simulink model "Hand"  (R2023b)
settings: Solver=ode45  StartTime=0.0  StopTime=100  RelTol=1e-3  EnableMultiTasking=on
model workspace (MAT data in the model file):
  InitialAngle = 0
libraries: simulink x22, vrlib x16, sharedtransform x15
(part 1 of 2)
Description:
  | Simulink(R) 3D Animation(TM) - Tutorial #3
  | 
  | Tutorial model to be used for 3D World Editor authoring example in the documentation.
  | After creating the virtual world according to the instructions in the documentation, include the VR block
  | in the model and connect B1, B2 coordinates and S scaling to corresponding nodes in
  | the virtual world.
settings Model: Creator=The MathWorks, Inc.  LastModifiedBy=25168
settings SolverCC: AlgebraicLoopSolver=TrustRegion
settings DataIOCC: LimitDataPoints=on  SaveFormat=Array  SaveOutput=off  SaveTime=off  ReturnWorkspaceOutputs=off  SignalLoggingName=logsOut
settings OptimizationCC: BooleanDataType=off  ExpressionDepthLimit=2147483647  InitFltsAndDblsToZero=on  LifeSpan=inf
settings DebuggingCC: UnderspecifiedInitializationDetection=Classic  MergeDetectMultiDrivingBlocksExec=none  CheckExecutionContextPreStartOutputMsg=on  SignalResolutionControl=TryResolveAllWithWarning  MultiTaskDSMMsg=warning  MultiTaskCondExecSysMsg=none  FcnCallInpInsideContextMsg=warning  UnconnectedInputMsg=warning  UnconnectedOutputMsg=warning  UnconnectedLineMsg=warning  StateNameClashWarn=warning  SymbolicDimsDataTypeCodeGenerationDiagnostic=none  SFUnexpectedBacktrackingDiag=warning  SFNoUnconditionalDefaultTransitionDiag=warning  SFExecutionAtInitializationDiag=none  ArithmeticOperatorsInVariantConditions=warning
settings HardwareCC: ProdBitPerPointer=32  ProdBitPerSizeT=32  ProdBitPerPtrDiffT=32  ProdLargestAtomicFloat=None  ProdIntDivRoundTo=Undefined  ProdEndianess=Unspecified  ProdWordSize=32  ProdHWDeviceType=32-bit Generic  TargetUnknown=on
settings ModelReferenceCC: UpdateModelReferenceTargets=IfOutOfDate  EnableRefExpFcnMdlSchedulingChecks=on  PropagateSignalLabelsOutOfModel=off
settings SFSimCC: SimUseLocalCustomCode=off  CustomCodeUndefinedFunction=UseInterfaceOnly
settings RTWCC: RTWUseLocalCustomCode=off
settings CodeAppCC: StateflowObjectComments=on
settings GRTTargetCC: TargetFcnLib=ansi_tfl_tmw.mat  TargetLangStandard=C89/C90 (ANSI)  CombineOutputUpdateFcns=off  GRTInterface=on
settings ConfigComp: CovMetricSettings=d  CovSaveCumulativeToWorkspaceVar=on  CovSaveSingleToWorkspaceVar=on  CovExternalEMLEnable=off  CovSFcnEnable=off

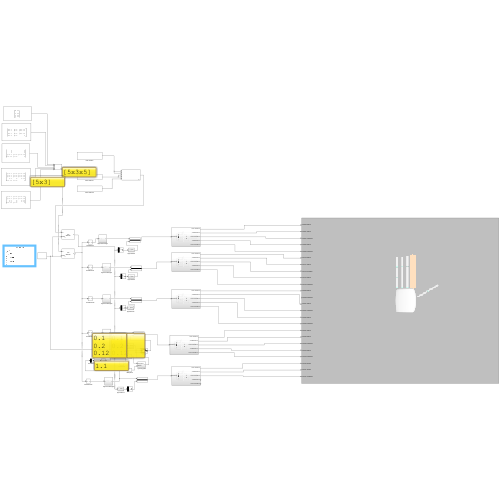
[thumbnail: Simulink's stored preview of the top-level diagram]
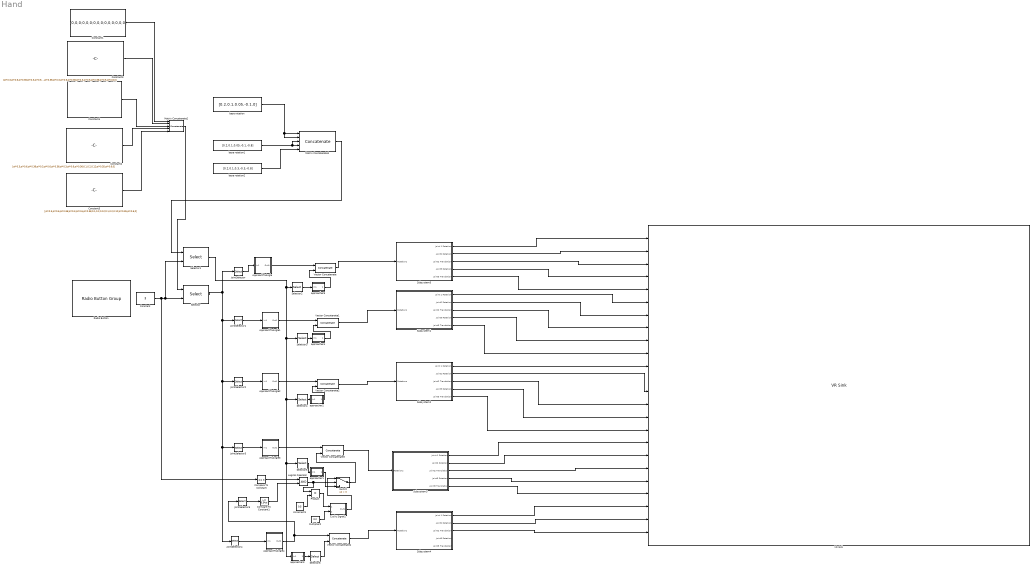
== system Hand ==
  ApproachToAngle : Subsystem
  ApproachToAngle1 : Subsystem
  ApproachToAngle2 : Subsystem
  ApproachToAngle3 : Subsystem
  ApproachToAngle4 : Subsystem
  Compare To Constant : simulink/Logic and Bit Operations/Compare To Constant  relop===  const=3  OutDataTypeStr=boolean
  Compare To Constant1 : simulink/Logic and Bit Operations/Compare To Constant  relop=>=  const=0.3*pi  OutDataTypeStr=boolean
  Constant : Constant  Value=3  VectorParams1D=off
  Constant1 : Constant  Value=[0,0,0;0,0,0;0,0,0;0,0,0;0,0,0]  VectorParams1D=off
  Constant2 : Constant  Value=[pi*0.3,pi*0.6,pi*0.36;pi*0.3,pi*0.6,pi*0.36;pi*0.3,pi*0.6,pi*0.36;0.1,0.2,0.12;pi*0.35,pi*0.6,0]  VectorParams1D=off
  Constant3 : Constant  Value=[pi*0.3,pi*0.6,pi*0.36;pi*0.3,pi*0.6,pi*0.36;pi*0.3,pi*0.6,pi*0.36;pi*0.3,pi*0.6,pi*0.36;pi*0.5,pi*0.8,0]  VectorParams1D=off
  Constant4 : Constant  Value=[0,0,0,;0,0,0;0,0,0;pi*0.1,pi*0.6,pi*0.36;pi*0.35,pi*0.6,0]  VectorParams1D=off
  Constant5 : Constant  Value=[pi*0.3,pi*0.6,pi*0.36;pi*0.3,pi*0.6,pi*0.36;0.1,0.2,0.12;0.1,0.2,0.12;pi*0.35,pi*0.6,0]  VectorParams1D=off
  Cyclic Signal2 : Subsystem
  JointSelector : Selector  NumberOfDimensions=2  IndexMode=Zero-based  InputPortWidth=3  IndexOptions=Index vector (dialog),Select all  Indices=0,0  OutputSizes=1,1
  JointSelector1 : Selector  NumberOfDimensions=2  IndexMode=Zero-based  InputPortWidth=3  IndexOptions=Index vector (dialog),Select all  Indices=1,1  OutputSizes=1,1
  JointSelector2 : Selector  NumberOfDimensions=2  IndexMode=Zero-based  InputPortWidth=3  IndexOptions=Index vector (dialog),Select all  Indices=2,2  OutputSizes=1,1
  JointSelector3 : Selector  NumberOfDimensions=2  IndexMode=Zero-based  InputPortWidth=3  IndexOptions=Index vector (dialog),Select all  Indices=3,2  OutputSizes=1,1
  JointSelector4 : Selector  NumberOfDimensions=2  IndexMode=Zero-based  InputPortWidth=3  IndexOptions=Index vector (dialog),Select all  Indices=4,2  OutputSizes=1,1
  JointSelector5 : Selector  IndexMode=Zero-based  InputPortWidth=3  IndexOptions=Index vector (dialog)  Indices=0  OutputSizes=1
  Logical Operator : Logic  AllPortsSameDT=off  OutDataTypeStr=boolean
  Matrix Concatenate1 : Concatenate  NumInputs=5  Mode=Multidimensional array  ConcatenateDimension=2
  Matrix Concatenate2 : Concatenate  NumInputs=5  Mode=Multidimensional array  ConcatenateDimension=3
  Multiplier2 : Constant  Value=0.2
  Product : Product
  Radio Button : RadioButtonGroup  SelectedLabel=No  ButtonGroupName=Group
      settings: Values={{'Open', 'Close', 'Pinch', 'No', 'V'}, [0 1 2 3 4]}
  Selector : Selector  NumberOfDimensions=3  IndexMode=Zero-based  InputPortWidth=3  IndexOptions=Select all,Select all,Starting index (port)  Indices=[1 3],1,1  OutputSizes=1,1,1
  Selector1 : Selector  NumberOfDimensions=2  IndexMode=Zero-based  InputPortWidth=3  IndexOptions=Select all,Index vector (port)  Indices=[1 3],1  OutputSizes=1,1
  Selector2 : Selector  IndexMode=Zero-based  InputPortWidth=5  IndexOptions=Index vector (dialog)  Indices=0  OutputSizes=1
  Selector3 : Selector  IndexMode=Zero-based  InputPortWidth=5  IndexOptions=Index vector (dialog)  Indices=1  OutputSizes=1
  Selector4 : Selector  IndexMode=Zero-based  InputPortWidth=5  IndexOptions=Index vector (dialog)  Indices=2  OutputSizes=1
  Selector5 : Selector  IndexMode=Zero-based  InputPortWidth=5  IndexOptions=Index vector (dialog)  Indices=3  OutputSizes=1
  Selector6 : Selector  IndexMode=Zero-based  InputPortWidth=5  IndexOptions=Index vector (dialog)  Indices=4  OutputSizes=1
  Subsystem1 : Subsystem
  Subsystem2 : Subsystem
  Subsystem3 : Subsystem
  Subsystem4 : Subsystem
  Subsystem5 : Subsystem
  Switch : Switch  Criteria=u2 > Threshold  ZeroCross=off  SaturateOnIntegerOverflow=off  InputSameDT=off
  VR Sink : vrlib/VR Sink  InstantiateOnLoad=on  SampleTime=0.1  ViewEnable=on  RemoteChange=off  RemoteView=off  FieldsWritten=Joint00.rotation.4.1.1.double#Joint01.rotation.4.1.1.double#Joint01.translation.3.1.1.double#Joint02.rotation.4.1.1.double#Joint02.translation.3.1.1.double#Joint10.rotation.4.1.1.double#Joint11.rotation.4.1.1.double#Joint11.translation.3.1.1.double#Joint12.rotation.4.1.1.double#Joint12.translation.3.1.1.double#Joint20.rotation.4.1.1.double#Joint20.translation.3.1.1.double#Joint21.rotation.4.1.1.double#Joint21.translation.3.1.1.double#Joint22.rotation.4.1.1.double#Joint22.translation.3.1.1.double#Joint31.rotation.4.1.1.double#Joint32.rotation.4.1.1.double#Joint32.translation.3.1.1.double#Joint33.rotation.4.1.1.double#Joint33.translation.3.1.1.double#JointT0.rotation.4.1.1.double#JointT1.rotation.4.1.1.double#JointT1.translation.3.1.1.double  WorldFileName=HW.x3d  AutoView=off  VideoDimensions=[]  AllowVariableSize=off  FigureProperties="{'Position', 'Name', 'Viewpoint', 'CameraBound', 'CameraDirection', 'CameraPosition', 'CameraUpVector', 'ZoomFactor', 'Antialiasing', 'Headlight', 'Lighting', 'NavPanel', 'Sound', 'StatusBar', 'Stereo3D', 'Stereo3DCameraOffset', 'Stereo3DHIT', 'ToolBar', 'Textures', 'Transparency', 'Triad', 'Wireframe', 'NavZones', 'NavMode', 'NavSpeed', 'CaptureFileFormat', 'CaptureFileName', 'Record2DCompressMethod', 'Record2DCompressQuality', 'Record2D', 'Record2DFileName', 'Record2DFPS'; [6.5500000000000000e+02   3.1433333333333337e+02   5.0933333333333326e+02   3.5000000000000000e+02], '', '', 'on', [-4.8608255793823621e-02  -6.0845975116805943e-02  -9.9696289037315999e-01], [9.6584636817473193e+00  -6.5460684286128101e-01   1.1919806951157568e+02], [4.8294533019942611e-02   9.9683214525226260e-01  -6.3192659956020442e-02], [1.0000000000000000e+00], 'on', 'on', 'on', 'halfbar', 'on', 'on', 'off', [1.0000000149011612e-01], [0.0000000000000000e+00], 'on', 'on', 'on', 'none', 'off', 'off', 'examine', 'normal', 'tif', '%f_anim_%n.tif', 'auto', [7.5000000000000000e+01], 'off', '%f_anim_%n.avi', 'auto'}"
  Vector Concatenate{,1..4} (5 alike) : Concatenate
  approacher1 : Subsystem
  approacher2 : Subsystem
  approacher3 : Subsystem
  approacher4 : Subsystem
  approacher5 : Subsystem
  base rotation : Constant  Value=[0.2,0.1,0.05,-0.1,0]
  base rotation1 : Constant  Value=[0.2,0.1,0.05,-0.1,-0.8]
  base rotation2 : Constant  Value=[0.2,0.1,0.3,-0.3,-0.8]
  increment1 : Constant  Value=0.5
  wires:
  Subsystem5/3(Joint2 Translation) -> VR Sink/3
  Subsystem5/4(Joint3 Rotation) -> VR Sink/4
  Subsystem5/1(Joint 1 Rotation) -> VR Sink/1
  Subsystem5/2(Joint2 Rotation) -> VR Sink/2
  Subsystem5/5(Joint3 Translation) -> VR Sink/5
  Subsystem1/1(Joint 1 Rotation) -> VR Sink/6
  Subsystem1/2(Joint2 Rotation) -> VR Sink/7
  Subsystem1/3(Joint2 Translation) -> VR Sink/8
  Subsystem1/4(Joint3 Rotation) -> VR Sink/9
  Subsystem1/5(Joint3 Translation) -> VR Sink/10
  Subsystem4/1(Joint 1 Rotation) -> VR Sink/22
  Subsystem4/2(Joint2 Rotation) -> VR Sink/23
  Subsystem4/3(Joint2 Translation) -> VR Sink/24
  Subsystem2/1(Joint 1 Rotation) -> VR Sink/11
  Subsystem2/2(Joint2 Rotation) -> VR Sink/13
  Subsystem2/3(Joint2 Translation) -> VR Sink/14
  Subsystem2/4(Joint3 Rotation) -> VR Sink/15
  Subsystem2/5(Joint3 Translation) -> VR Sink/16
  Subsystem3/1(Joint 1 Rotation) -> VR Sink/17
  Subsystem3/2(Joint2 Rotation) -> VR Sink/18
  Subsystem3/3(Joint2 Translation) -> VR Sink/19
  Subsystem3/4(Joint3 Rotation) -> VR Sink/20
  Subsystem3/5(Joint3 Translation) -> VR Sink/21
  Constant/1 -> Compare To Constant/1, Selector1/2, Selector/2
  Constant1/1 -> Matrix Concatenate2/1
  Constant2/1 -> Matrix Concatenate2/4
  Constant3/1 -> Matrix Concatenate2/2
  Matrix Concatenate2/1 -> Selector/1
  ApproachToAngle/1(Out1) -> Vector Concatenate/1
  JointSelector/1 -> ApproachToAngle/1(In1)
  JointSelector2/1 -> ApproachToAngle2/1(In1)
  Selector/1 -> JointSelector1/1, JointSelector4/1, JointSelector3/1, JointSelector2/1, JointSelector/1
  Vector Concatenate/1 -> Subsystem5/1(Rotations)
  ApproachToAngle1/1(Out1) -> Vector Concatenate1/1
  JointSelector1/1 -> ApproachToAngle1/1(In1)
  Vector Concatenate1/1 -> Subsystem1/1(Rotations)
  ApproachToAngle2/1(Out1) -> Vector Concatenate2/1
  Selector4/1 -> approacher2/1(In1)
  Vector Concatenate2/1 -> Subsystem2/1(Rotations)
  ApproachToAngle3/1(Out1) -> Vector Concatenate3/1
  JointSelector3/1 -> ApproachToAngle3/1(In1)
  ApproachToAngle4/1(Out1) -> JointSelector5/1, Vector Concatenate4/1
  Selector6/1 -> Vector Concatenate4/2
  JointSelector4/1 -> ApproachToAngle4/1(In1)
  Vector Concatenate4/1 -> Subsystem4/1(Rotations)
  Selector1/1 -> approacher3/1(In1), Selector5/1, Selector4/1, Selector3/1, Selector2/1
  base rotation/1 -> Matrix Concatenate1/2, Matrix Concatenate1/1
  base rotation1/1 -> Matrix Concatenate1/3, Matrix Concatenate1/4
  Constant4/1 -> Matrix Concatenate2/3
  Matrix Concatenate1/1 -> Selector1/1
  Compare To Constant/1 -> Logical Operator/1
  Multiplier2/1 -> Cyclic Signal2/2(Scaler)
  increment1/1 -> Product/2
  Logical Operator/1 -> Product/1, Switch/2
  JointSelector5/1 -> Compare To Constant1/1
  Constant5/1 -> Matrix Concatenate2/5
  Vector Concatenate3/1 -> Subsystem3/1(Rotations)
  Switch/1 -> Vector Concatenate3/2
  Cyclic Signal2/1(Out1) -> Switch/1
  Compare To Constant1/1 -> Logical Operator/2
  Product/1 -> Cyclic Signal2/1(Frequency)
  base rotation2/1 -> Matrix Concatenate1/5
  approacher3/1(Joint 1) -> Selector6/1
  Selector5/1 -> approacher1/1(In1)
  approacher1/1(Joint 1) -> Switch/3
  approacher2/1(Joint 1) -> Vector Concatenate2/2
  Selector3/1 -> approacher4/1(In1)
  approacher4/1(Joint 1) -> Vector Concatenate1/2
  Selector2/1 -> approacher5/1(In1)
  approacher5/1(Joint 1) -> Vector Concatenate/2

== system Hand/ApproachToAngle ==
  In1 : Inport
  Matrix Concatenate1 : Concatenate  NumInputs=3  ConcatenateDimension=2
  Selector1 : Selector  IndexMode=Zero-based  InputPortWidth=3  IndexOptions=Index vector (dialog)  Indices=1  OutputSizes=1
  Selector2 : Selector  IndexMode=Zero-based  InputPortWidth=3  IndexOptions=Index vector (dialog)  Indices=0  OutputSizes=1  RuntimeRangeChecks=on
  Selector3 : Selector  IndexMode=Zero-based  InputPortWidth=3  IndexOptions=Index vector (dialog)  Indices=2  OutputSizes=1
  approacher1 : Subsystem
  approacher2 : Subsystem
  approacher3 : Subsystem
  Out1 : Outport
  wires:
  Selector3/1 -> approacher3/1(In1)
  Selector2/1 -> approacher2/1(In1)
  approacher3/1(Joint 1) -> Matrix Concatenate1/3
  approacher1/1(Joint 1) -> Matrix Concatenate1/2
  approacher2/1(Joint 1) -> Matrix Concatenate1/1
  Selector1/1 -> approacher1/1(In1)
  In1/1 -> Selector3/1, Selector2/1, Selector1/1
  Matrix Concatenate1/1 -> Out1/1

== system Hand/ApproachToAngle1 ==
  In1 : Inport
  Matrix Concatenate1 : Concatenate  NumInputs=3  ConcatenateDimension=2
  Selector1 : Selector  IndexMode=Zero-based  InputPortWidth=3  IndexOptions=Index vector (dialog)  Indices=1  OutputSizes=1
  Selector2 : Selector  IndexMode=Zero-based  InputPortWidth=3  IndexOptions=Index vector (dialog)  Indices=0  OutputSizes=1  RuntimeRangeChecks=on
  Selector3 : Selector  IndexMode=Zero-based  InputPortWidth=3  IndexOptions=Index vector (dialog)  Indices=2  OutputSizes=1
  approacher1 : Subsystem
  approacher2 : Subsystem
  approacher3 : Subsystem
  Out1 : Outport
  wires:
  Selector3/1 -> approacher3/1(In1)
  Selector2/1 -> approacher2/1(In1)
  approacher3/1(Joint 1) -> Matrix Concatenate1/3
  approacher1/1(Joint 1) -> Matrix Concatenate1/2
  approacher2/1(Joint 1) -> Matrix Concatenate1/1
  Selector1/1 -> approacher1/1(In1)
  In1/1 -> Selector3/1, Selector2/1, Selector1/1
  Matrix Concatenate1/1 -> Out1/1

== system Hand/ApproachToAngle2 ==
  In1 : Inport
  Matrix Concatenate1 : Concatenate  NumInputs=3  ConcatenateDimension=2
  Selector1 : Selector  IndexMode=Zero-based  InputPortWidth=3  IndexOptions=Index vector (dialog)  Indices=1  OutputSizes=1
  Selector2 : Selector  IndexMode=Zero-based  InputPortWidth=3  IndexOptions=Index vector (dialog)  Indices=0  OutputSizes=1  RuntimeRangeChecks=on
  Selector3 : Selector  IndexMode=Zero-based  InputPortWidth=3  IndexOptions=Index vector (dialog)  Indices=2  OutputSizes=1
  approacher1 : Subsystem
  approacher2 : Subsystem
  approacher3 : Subsystem
  Out1 : Outport
  wires:
  Selector3/1 -> approacher3/1(In1)
  Selector2/1 -> approacher2/1(In1)
  approacher3/1(Joint 1) -> Matrix Concatenate1/3
  approacher1/1(Joint 1) -> Matrix Concatenate1/2
  approacher2/1(Joint 1) -> Matrix Concatenate1/1
  Selector1/1 -> approacher1/1(In1)
  In1/1 -> Selector3/1, Selector2/1, Selector1/1
  Matrix Concatenate1/1 -> Out1/1

== system Hand/ApproachToAngle3 ==
  In1 : Inport
  Matrix Concatenate1 : Concatenate  NumInputs=3  ConcatenateDimension=2
  Selector1 : Selector  IndexMode=Zero-based  InputPortWidth=3  IndexOptions=Index vector (dialog)  Indices=1  OutputSizes=1
  Selector2 : Selector  IndexMode=Zero-based  InputPortWidth=3  IndexOptions=Index vector (dialog)  Indices=0  OutputSizes=1  RuntimeRangeChecks=on
  Selector3 : Selector  IndexMode=Zero-based  InputPortWidth=3  IndexOptions=Index vector (dialog)  Indices=2  OutputSizes=1
  approacher1 : Subsystem
  approacher2 : Subsystem
  approacher3 : Subsystem
  Out1 : Outport
  wires:
  Selector3/1 -> approacher3/1(In1)
  Selector2/1 -> approacher2/1(In1)
  approacher3/1(Joint 1) -> Matrix Concatenate1/3
  approacher1/1(Joint 1) -> Matrix Concatenate1/2
  approacher2/1(Joint 1) -> Matrix Concatenate1/1
  Selector1/1 -> approacher1/1(In1)
  In1/1 -> Selector3/1, Selector2/1, Selector1/1
  Matrix Concatenate1/1 -> Out1/1

== system Hand/ApproachToAngle4 ==
  In1 : Inport
  Matrix Concatenate1 : Concatenate  NumInputs=3  ConcatenateDimension=2
  Selector1 : Selector  IndexMode=Zero-based  InputPortWidth=3  IndexOptions=Index vector (dialog)  Indices=1  OutputSizes=1
  Selector2 : Selector  IndexMode=Zero-based  InputPortWidth=3  IndexOptions=Index vector (dialog)  Indices=0  OutputSizes=1  RuntimeRangeChecks=on
  Selector3 : Selector  IndexMode=Zero-based  InputPortWidth=3  IndexOptions=Index vector (dialog)  Indices=2  OutputSizes=1
  approacher1 : Subsystem
  approacher2 : Subsystem
  approacher3 : Subsystem
  Out1 : Outport
  wires:
  Selector3/1 -> approacher3/1(In1)
  Selector2/1 -> approacher2/1(In1)
  approacher3/1(Joint 1) -> Matrix Concatenate1/3
  approacher1/1(Joint 1) -> Matrix Concatenate1/2
  approacher2/1(Joint 1) -> Matrix Concatenate1/1
  Selector1/1 -> approacher1/1(In1)
  In1/1 -> Selector3/1, Selector2/1, Selector1/1
  Matrix Concatenate1/1 -> Out1/1

== system Hand/Cyclic Signal2 ==
  Frequency : Inport
  Scaler : Inport  Port=2
  Constant : Constant  Value=pi
  Integrator : Integrator  UpperSaturationLimit=Inf  LowerSaturationLimit=-Inf
  Product : Product
  Product1 : Product
  Trigonometric Function5 : Trigonometry
  Out1 : Outport
  wires:
  Integrator/1 -> Trigonometric Function5/1
  Trigonometric Function5/1 -> Product1/1
  Product1/1 -> Out1/1
  Scaler/1 -> Product1/2
  Frequency/1 -> Product/1
  Constant/1 -> Product/2
  Product/1 -> Integrator/1

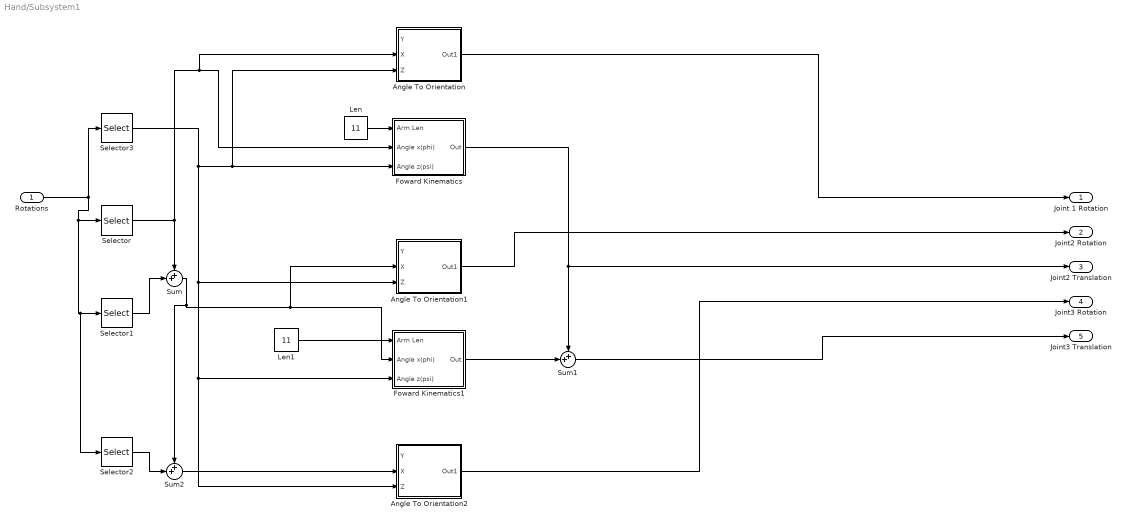
== system Hand/Subsystem1 ==
  Rotations : Inport
  Angle To Orientation : Subsystem
  Angle To Orientation1 : Subsystem
  Angle To Orientation2 : Subsystem
  Foward Kinematics : Subsystem
  Foward Kinematics1 : Subsystem
  Len : Constant  Value=11
  Len1 : Constant  Value=11
  Selector : Selector  InputPortWidth=4  IndexOptions=Index vector (dialog)  Indices=1  OutputSizes=1
  Selector1 : Selector  InputPortWidth=4  IndexOptions=Index vector (dialog)  Indices=2  OutputSizes=1
  Selector2 : Selector  InputPortWidth=4  IndexOptions=Index vector (dialog)  Indices=3  OutputSizes=1
  Selector3 : Selector  InputPortWidth=4  IndexOptions=Index vector (dialog)  Indices=4  OutputSizes=1
  Sum : Sum  Inputs=++|
  Sum1 : Sum  Inputs=++|
  Sum2 : Sum  Inputs=++|
  Joint 1 Rotation : Outport
  Joint2 Rotation : Outport  Port=2
  Joint2 Translation : Outport  Port=3
  Joint3 Rotation : Outport  Port=4
  Joint3 Translation : Outport  Port=5
  wires:
  Foward Kinematics/1(Out) -> Joint2 Translation/1, Sum1/1
  Selector3/1 -> Foward Kinematics1/3(Angle z(psi)), Angle To Orientation2/3(Z), Angle To Orientation1/3(Z), Angle To Orientation/3(Z), Foward Kinematics/3(Angle z(psi))
  Sum2/1 -> Angle To Orientation2/2(X)
  Selector/1 -> Angle To Orientation/2(X), Foward Kinematics/2(Angle x(phi)), Sum/1
  Sum1/1 -> Joint3 Translation/1
  Sum/1 -> Sum2/1, Angle To Orientation1/2(X), Foward Kinematics1/2(Angle x(phi))
  Len/1 -> Foward Kinematics/1(Arm Len)
  Foward Kinematics1/1(Out) -> Sum1/2
  Len1/1 -> Foward Kinematics1/1(Arm Len)
  Angle To Orientation1/1(Out1) -> Joint2 Rotation/1
  Angle To Orientation2/1(Out1) -> Joint3 Rotation/1
  Angle To Orientation/1(Out1) -> Joint 1 Rotation/1
  Selector2/1 -> Sum2/2
  Selector1/1 -> Sum/2
  Rotations/1 -> Selector2/1, Selector1/1, Selector/1, Selector3/1

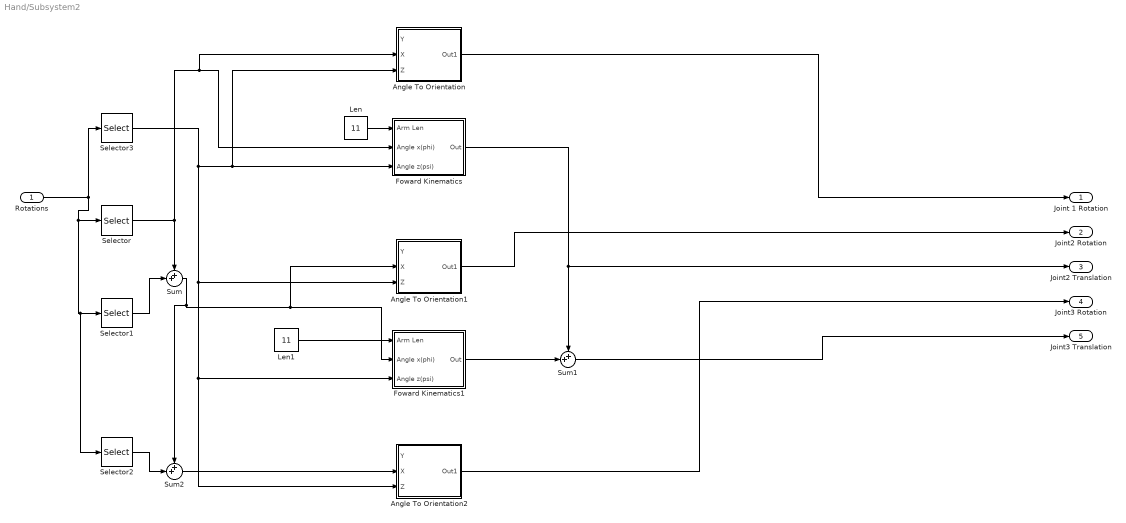
== system Hand/Subsystem2 ==
  Rotations : Inport
  Angle To Orientation : Subsystem
  Angle To Orientation1 : Subsystem
  Angle To Orientation2 : Subsystem
  Foward Kinematics : Subsystem
  Foward Kinematics1 : Subsystem
  Len : Constant  Value=11
  Len1 : Constant  Value=11
  Selector : Selector  InputPortWidth=4  IndexOptions=Index vector (dialog)  Indices=1  OutputSizes=1
  Selector1 : Selector  InputPortWidth=4  IndexOptions=Index vector (dialog)  Indices=2  OutputSizes=1
  Selector2 : Selector  InputPortWidth=4  IndexOptions=Index vector (dialog)  Indices=3  OutputSizes=1
  Selector3 : Selector  InputPortWidth=4  IndexOptions=Index vector (dialog)  Indices=4  OutputSizes=1
  Sum : Sum  Inputs=++|
  Sum1 : Sum  Inputs=++|
  Sum2 : Sum  Inputs=++|
  Joint 1 Rotation : Outport
  Joint2 Rotation : Outport  Port=2
  Joint2 Translation : Outport  Port=3
  Joint3 Rotation : Outport  Port=4
  Joint3 Translation : Outport  Port=5
  wires:
  Foward Kinematics/1(Out) -> Joint2 Translation/1, Sum1/1
  Selector3/1 -> Foward Kinematics1/3(Angle z(psi)), Angle To Orientation2/3(Z), Angle To Orientation1/3(Z), Angle To Orientation/3(Z), Foward Kinematics/3(Angle z(psi))
  Sum2/1 -> Angle To Orientation2/2(X)
  Selector/1 -> Angle To Orientation/2(X), Foward Kinematics/2(Angle x(phi)), Sum/1
  Sum1/1 -> Joint3 Translation/1
  Sum/1 -> Sum2/1, Angle To Orientation1/2(X), Foward Kinematics1/2(Angle x(phi))
  Len/1 -> Foward Kinematics/1(Arm Len)
  Foward Kinematics1/1(Out) -> Sum1/2
  Len1/1 -> Foward Kinematics1/1(Arm Len)
  Angle To Orientation1/1(Out1) -> Joint2 Rotation/1
  Angle To Orientation2/1(Out1) -> Joint3 Rotation/1
  Angle To Orientation/1(Out1) -> Joint 1 Rotation/1
  Selector2/1 -> Sum2/2
  Selector1/1 -> Sum/2
  Rotations/1 -> Selector2/1, Selector1/1, Selector/1, Selector3/1

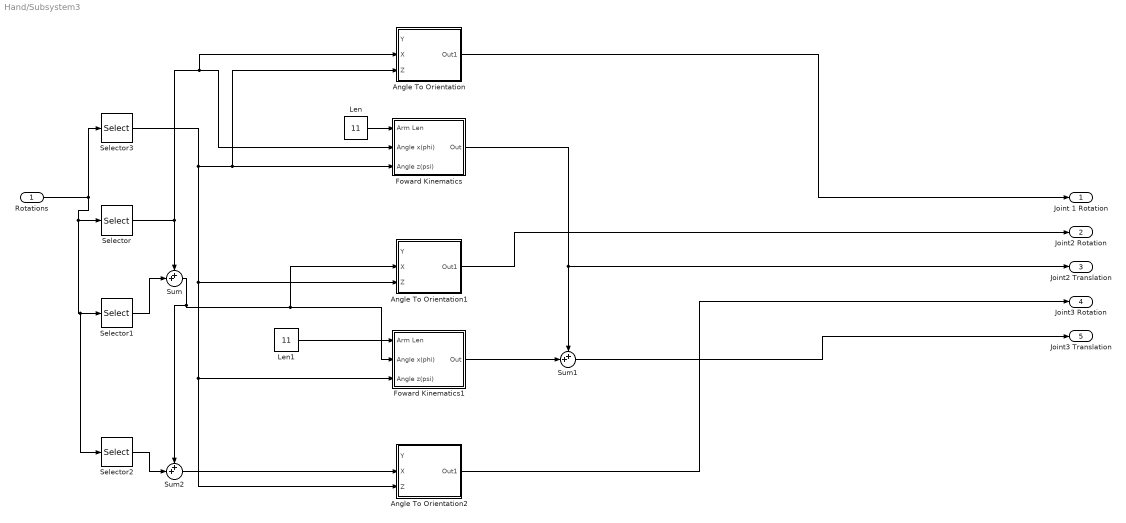
== system Hand/Subsystem3 ==
  Rotations : Inport
  Angle To Orientation : Subsystem
  Angle To Orientation1 : Subsystem
  Angle To Orientation2 : Subsystem
  Foward Kinematics : Subsystem
  Foward Kinematics1 : Subsystem
  Len : Constant  Value=11
  Len1 : Constant  Value=11
  Selector : Selector  InputPortWidth=4  IndexOptions=Index vector (dialog)  Indices=1  OutputSizes=1
  Selector1 : Selector  InputPortWidth=4  IndexOptions=Index vector (dialog)  Indices=2  OutputSizes=1
  Selector2 : Selector  InputPortWidth=4  IndexOptions=Index vector (dialog)  Indices=3  OutputSizes=1
  Selector3 : Selector  InputPortWidth=4  IndexOptions=Index vector (dialog)  Indices=4  OutputSizes=1
  Sum : Sum  Inputs=++|
  Sum1 : Sum  Inputs=++|
  Sum2 : Sum  Inputs=++|
  Joint 1 Rotation : Outport
  Joint2 Rotation : Outport  Port=2
  Joint2 Translation : Outport  Port=3
  Joint3 Rotation : Outport  Port=4
  Joint3 Translation : Outport  Port=5
  wires:
  Foward Kinematics/1(Out) -> Joint2 Translation/1, Sum1/1
  Selector3/1 -> Foward Kinematics1/3(Angle z(psi)), Angle To Orientation2/3(Z), Angle To Orientation1/3(Z), Angle To Orientation/3(Z), Foward Kinematics/3(Angle z(psi))
  Sum2/1 -> Angle To Orientation2/2(X)
  Selector/1 -> Angle To Orientation/2(X), Foward Kinematics/2(Angle x(phi)), Sum/1
  Sum1/1 -> Joint3 Translation/1
  Sum/1 -> Sum2/1, Angle To Orientation1/2(X), Foward Kinematics1/2(Angle x(phi))
  Len/1 -> Foward Kinematics/1(Arm Len)
  Foward Kinematics1/1(Out) -> Sum1/2
  Len1/1 -> Foward Kinematics1/1(Arm Len)
  Angle To Orientation1/1(Out1) -> Joint2 Rotation/1
  Angle To Orientation2/1(Out1) -> Joint3 Rotation/1
  Angle To Orientation/1(Out1) -> Joint 1 Rotation/1
  Selector2/1 -> Sum2/2
  Selector1/1 -> Sum/2
  Rotations/1 -> Selector2/1, Selector1/1, Selector/1, Selector3/1

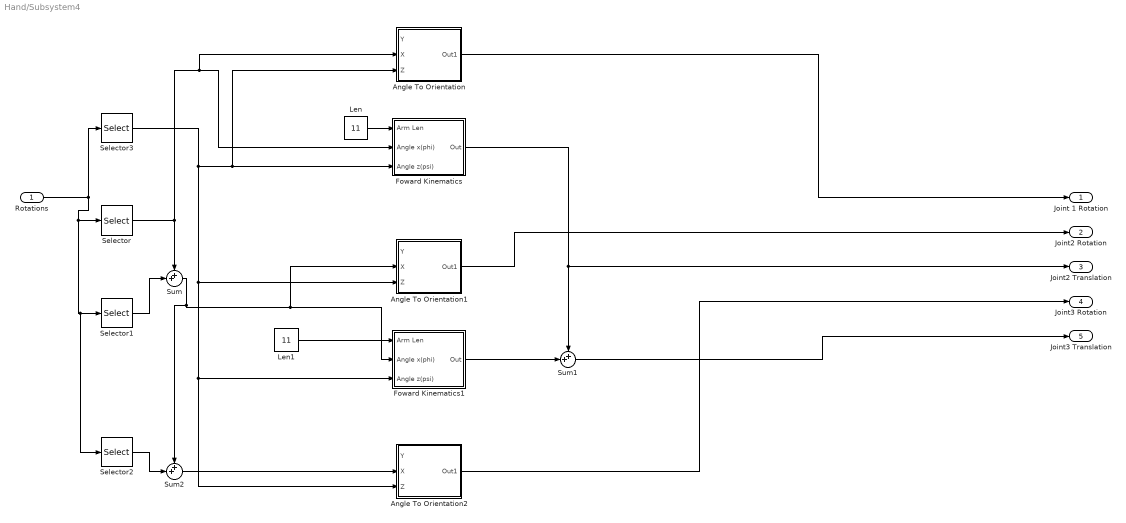
== system Hand/Subsystem4 ==
  Rotations : Inport
  Angle To Orientation : Subsystem
  Angle To Orientation1 : Subsystem
  Angle To Orientation2 : Subsystem
  Foward Kinematics : Subsystem
  Foward Kinematics1 : Subsystem
  Len : Constant  Value=11
  Len1 : Constant  Value=11
  Selector : Selector  InputPortWidth=4  IndexOptions=Index vector (dialog)  Indices=1  OutputSizes=1
  Selector1 : Selector  InputPortWidth=4  IndexOptions=Index vector (dialog)  Indices=2  OutputSizes=1
  Selector2 : Selector  InputPortWidth=4  IndexOptions=Index vector (dialog)  Indices=3  OutputSizes=1
  Selector3 : Selector  InputPortWidth=4  IndexOptions=Index vector (dialog)  Indices=4  OutputSizes=1
  Sum : Sum  Inputs=++|
  Sum1 : Sum  Inputs=++|
  Sum2 : Sum  Inputs=++|
  Joint 1 Rotation : Outport
  Joint2 Rotation : Outport  Port=2
  Joint2 Translation : Outport  Port=3
  Joint3 Rotation : Outport  Port=4
  Joint3 Translation : Outport  Port=5
  wires:
  Foward Kinematics/1(Out) -> Joint2 Translation/1, Sum1/1
  Selector3/1 -> Foward Kinematics1/3(Angle z(psi)), Angle To Orientation2/3(Z), Angle To Orientation1/3(Z), Angle To Orientation/3(Z), Foward Kinematics/3(Angle z(psi))
  Sum2/1 -> Angle To Orientation2/2(X)
  Selector/1 -> Angle To Orientation/2(X), Foward Kinematics/2(Angle x(phi)), Sum/1
  Sum1/1 -> Joint3 Translation/1
  Sum/1 -> Sum2/1, Angle To Orientation1/2(X), Foward Kinematics1/2(Angle x(phi))
  Len/1 -> Foward Kinematics/1(Arm Len)
  Foward Kinematics1/1(Out) -> Sum1/2
  Len1/1 -> Foward Kinematics1/1(Arm Len)
  Angle To Orientation1/1(Out1) -> Joint2 Rotation/1
  Angle To Orientation2/1(Out1) -> Joint3 Rotation/1
  Angle To Orientation/1(Out1) -> Joint 1 Rotation/1
  Selector2/1 -> Sum2/2
  Selector1/1 -> Sum/2
  Rotations/1 -> Selector2/1, Selector1/1, Selector/1, Selector3/1

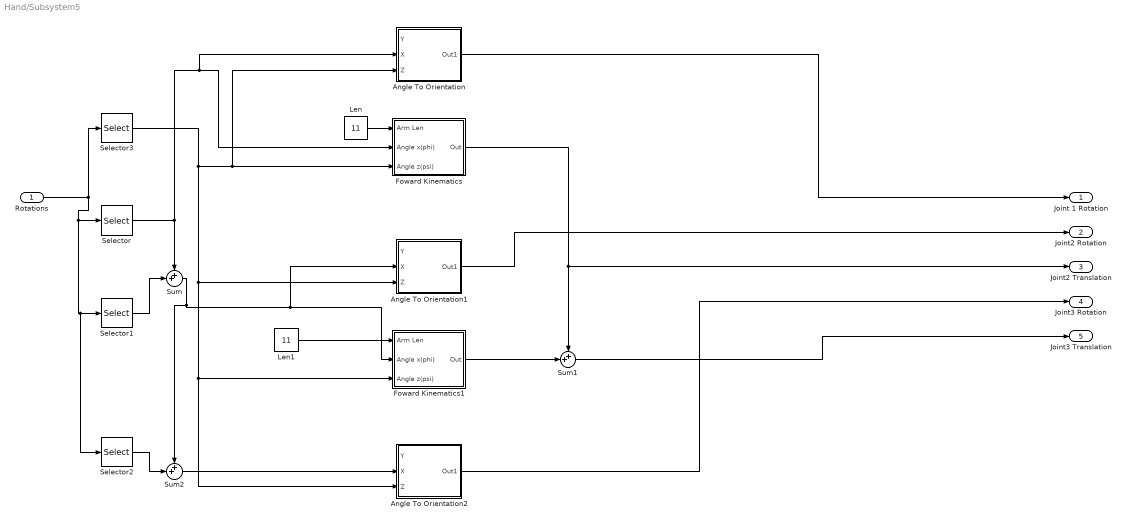
== system Hand/Subsystem5 ==
  Rotations : Inport
  Angle To Orientation : Subsystem
  Angle To Orientation1 : Subsystem
  Angle To Orientation2 : Subsystem
  Foward Kinematics : Subsystem
  Foward Kinematics1 : Subsystem
  Len : Constant  Value=11
  Len1 : Constant  Value=11
  Selector : Selector  InputPortWidth=4  IndexOptions=Index vector (dialog)  Indices=1  OutputSizes=1
  Selector1 : Selector  InputPortWidth=4  IndexOptions=Index vector (dialog)  Indices=2  OutputSizes=1
  Selector2 : Selector  InputPortWidth=4  IndexOptions=Index vector (dialog)  Indices=3  OutputSizes=1
  Selector3 : Selector  InputPortWidth=4  IndexOptions=Index vector (dialog)  Indices=4  OutputSizes=1
  Sum : Sum  Inputs=++|
  Sum1 : Sum  Inputs=++|
  Sum2 : Sum  Inputs=++|
  Joint 1 Rotation : Outport
  Joint2 Rotation : Outport  Port=2
  Joint2 Translation : Outport  Port=3
  Joint3 Rotation : Outport  Port=4
  Joint3 Translation : Outport  Port=5
  wires:
  Foward Kinematics/1(Out) -> Joint2 Translation/1, Sum1/1
  Selector3/1 -> Foward Kinematics1/3(Angle z(psi)), Angle To Orientation2/3(Z), Angle To Orientation1/3(Z), Angle To Orientation/3(Z), Foward Kinematics/3(Angle z(psi))
  Sum2/1 -> Angle To Orientation2/2(X)
  Selector/1 -> Angle To Orientation/2(X), Foward Kinematics/2(Angle x(phi)), Sum/1
  Sum1/1 -> Joint3 Translation/1
  Sum/1 -> Sum2/1, Angle To Orientation1/2(X), Foward Kinematics1/2(Angle x(phi))
  Len/1 -> Foward Kinematics/1(Arm Len)
  Foward Kinematics1/1(Out) -> Sum1/2
  Len1/1 -> Foward Kinematics1/1(Arm Len)
  Angle To Orientation1/1(Out1) -> Joint2 Rotation/1
  Angle To Orientation2/1(Out1) -> Joint3 Rotation/1
  Angle To Orientation/1(Out1) -> Joint 1 Rotation/1
  Selector2/1 -> Sum2/2
  Selector1/1 -> Sum/2
  Rotations/1 -> Selector2/1, Selector1/1, Selector/1, Selector3/1

== system Hand/approacher1 ==
  In1 : Inport
  Compare To Zero : simulink/Logic and Bit Operations/Compare To Zero  relop=<=  OutDataTypeStr=boolean  ZeroCross=off
  Gain : Gain  Gain=-1
  Integrator : Integrator  ZeroCross=off
  Subtract : Sum  Inputs=+-
  Switch : Switch  Criteria=u2 > Threshold  ZeroCross=off  SaturateOnIntegerOverflow=off  InputSameDT=off
  increment : Constant  Value=0.2
  Joint 1 : Outport
  wires:
  Gain/1 -> Switch/3
  Subtract/1 -> Compare To Zero/1
  Compare To Zero/1 -> Switch/2
  Integrator/1 -> Joint 1/1, Subtract/1
  Switch/1 -> Integrator/1
  increment/1 -> Switch/1, Gain/1
  In1/1 -> Subtract/2

== system Hand/approacher2 ==
  In1 : Inport
  Compare To Zero : simulink/Logic and Bit Operations/Compare To Zero  relop=<=  OutDataTypeStr=boolean  ZeroCross=off
  Gain : Gain  Gain=-1
  Integrator : Integrator  ZeroCross=off
  Subtract : Sum  Inputs=+-
  Switch : Switch  Criteria=u2 > Threshold  ZeroCross=off  SaturateOnIntegerOverflow=off  InputSameDT=off
  increment : Constant  Value=0.2
  Joint 1 : Outport
  wires:
  Gain/1 -> Switch/3
  Subtract/1 -> Compare To Zero/1
  Compare To Zero/1 -> Switch/2
  Integrator/1 -> Joint 1/1, Subtract/1
  Switch/1 -> Integrator/1
  increment/1 -> Switch/1, Gain/1
  In1/1 -> Subtract/2

== system Hand/approacher3 ==
  In1 : Inport
  Compare To Zero : simulink/Logic and Bit Operations/Compare To Zero  relop=<=  OutDataTypeStr=boolean  ZeroCross=off
  Gain : Gain  Gain=-1
  Integrator : Integrator  ZeroCross=off
  Subtract : Sum  Inputs=+-
  Switch : Switch  Criteria=u2 > Threshold  ZeroCross=off  SaturateOnIntegerOverflow=off  InputSameDT=off
  increment : Constant  Value=0.2
  Joint 1 : Outport
  wires:
  Gain/1 -> Switch/3
  Subtract/1 -> Compare To Zero/1
  Compare To Zero/1 -> Switch/2
  Integrator/1 -> Joint 1/1, Subtract/1
  Switch/1 -> Integrator/1
  increment/1 -> Switch/1, Gain/1
  In1/1 -> Subtract/2

== system Hand/approacher4 ==
  In1 : Inport
  Compare To Zero : simulink/Logic and Bit Operations/Compare To Zero  relop=<=  OutDataTypeStr=boolean  ZeroCross=off
  Gain : Gain  Gain=-1
  Integrator : Integrator  ZeroCross=off
  Subtract : Sum  Inputs=+-
  Switch : Switch  Criteria=u2 > Threshold  ZeroCross=off  SaturateOnIntegerOverflow=off  InputSameDT=off
  increment : Constant  Value=0.2
  Joint 1 : Outport
  wires:
  Gain/1 -> Switch/3
  Subtract/1 -> Compare To Zero/1
  Compare To Zero/1 -> Switch/2
  Integrator/1 -> Joint 1/1, Subtract/1
  Switch/1 -> Integrator/1
  increment/1 -> Switch/1, Gain/1
  In1/1 -> Subtract/2

== system Hand/approacher5 ==
  In1 : Inport
  Compare To Zero : simulink/Logic and Bit Operations/Compare To Zero  relop=<=  OutDataTypeStr=boolean  ZeroCross=off
  Gain : Gain  Gain=-1
  Integrator : Integrator  ZeroCross=off
  Subtract : Sum  Inputs=+-
  Switch : Switch  Criteria=u2 > Threshold  ZeroCross=off  SaturateOnIntegerOverflow=off  InputSameDT=off
  increment : Constant  Value=0.2
  Joint 1 : Outport
  wires:
  Gain/1 -> Switch/3
  Subtract/1 -> Compare To Zero/1
  Compare To Zero/1 -> Switch/2
  Integrator/1 -> Joint 1/1, Subtract/1
  Switch/1 -> Integrator/1
  increment/1 -> Switch/1, Gain/1
  In1/1 -> Subtract/2

== system Hand/ApproachToAngle/approacher1 ==
  In1 : Inport
  Compare To Zero : simulink/Logic and Bit Operations/Compare To Zero  relop=<=  OutDataTypeStr=boolean  ZeroCross=off
  Gain : Gain  Gain=-1
  Integrator : Integrator  ZeroCross=off
  Subtract : Sum  Inputs=+-
  Switch : Switch  Criteria=u2 > Threshold  ZeroCross=off  SaturateOnIntegerOverflow=off  InputSameDT=off
  increment : Constant  Value=0.2
  Joint 1 : Outport
  wires:
  Gain/1 -> Switch/3
  Subtract/1 -> Compare To Zero/1
  Compare To Zero/1 -> Switch/2
  Integrator/1 -> Joint 1/1, Subtract/1
  Switch/1 -> Integrator/1
  increment/1 -> Switch/1, Gain/1
  In1/1 -> Subtract/2

== system Hand/ApproachToAngle/approacher2 ==
  In1 : Inport
  Compare To Zero : simulink/Logic and Bit Operations/Compare To Zero  relop=<=  OutDataTypeStr=boolean  ZeroCross=off
  Gain : Gain  Gain=-1
  Integrator : Integrator  ZeroCross=off
  Subtract : Sum  Inputs=+-
  Switch : Switch  Criteria=u2 > Threshold  ZeroCross=off  SaturateOnIntegerOverflow=off  InputSameDT=off
  increment : Constant  Value=0.2
  Joint 1 : Outport
  wires:
  Gain/1 -> Switch/3
  Subtract/1 -> Compare To Zero/1
  Compare To Zero/1 -> Switch/2
  Integrator/1 -> Joint 1/1, Subtract/1
  Switch/1 -> Integrator/1
  increment/1 -> Switch/1, Gain/1
  In1/1 -> Subtract/2

== system Hand/ApproachToAngle/approacher3 ==
  In1 : Inport
  Compare To Zero : simulink/Logic and Bit Operations/Compare To Zero  relop=<=  OutDataTypeStr=boolean  ZeroCross=off
  Gain : Gain  Gain=-1
  Integrator : Integrator  ZeroCross=off
  Subtract : Sum  Inputs=+-
  Switch : Switch  Criteria=u2 > Threshold  ZeroCross=off  SaturateOnIntegerOverflow=off  InputSameDT=off
  increment : Constant  Value=0.2
  Joint 1 : Outport
  wires:
  Gain/1 -> Switch/3
  Subtract/1 -> Compare To Zero/1
  Compare To Zero/1 -> Switch/2
  Integrator/1 -> Joint 1/1, Subtract/1
  Switch/1 -> Integrator/1
  increment/1 -> Switch/1, Gain/1
  In1/1 -> Subtract/2

== system Hand/ApproachToAngle1/approacher1 ==
  In1 : Inport
  Compare To Zero : simulink/Logic and Bit Operations/Compare To Zero  relop=<=  OutDataTypeStr=boolean  ZeroCross=off
  Gain : Gain  Gain=-1
  Integrator : Integrator  ZeroCross=off
  Subtract : Sum  Inputs=+-
  Switch : Switch  Criteria=u2 > Threshold  ZeroCross=off  SaturateOnIntegerOverflow=off  InputSameDT=off
  increment : Constant  Value=0.2
  Joint 1 : Outport
  wires:
  Gain/1 -> Switch/3
  Subtract/1 -> Compare To Zero/1
  Compare To Zero/1 -> Switch/2
  Integrator/1 -> Joint 1/1, Subtract/1
  Switch/1 -> Integrator/1
  increment/1 -> Switch/1, Gain/1
  In1/1 -> Subtract/2

== system Hand/ApproachToAngle1/approacher2 ==
  In1 : Inport
  Compare To Zero : simulink/Logic and Bit Operations/Compare To Zero  relop=<=  OutDataTypeStr=boolean  ZeroCross=off
  Gain : Gain  Gain=-1
  Integrator : Integrator  ZeroCross=off
  Subtract : Sum  Inputs=+-
  Switch : Switch  Criteria=u2 > Threshold  ZeroCross=off  SaturateOnIntegerOverflow=off  InputSameDT=off
  increment : Constant  Value=0.2
  Joint 1 : Outport
  wires:
  Gain/1 -> Switch/3
  Subtract/1 -> Compare To Zero/1
  Compare To Zero/1 -> Switch/2
  Integrator/1 -> Joint 1/1, Subtract/1
  Switch/1 -> Integrator/1
  increment/1 -> Switch/1, Gain/1
  In1/1 -> Subtract/2

== system Hand/ApproachToAngle1/approacher3 ==
  In1 : Inport
  Compare To Zero : simulink/Logic and Bit Operations/Compare To Zero  relop=<=  OutDataTypeStr=boolean  ZeroCross=off
  Gain : Gain  Gain=-1
  Integrator : Integrator  ZeroCross=off
  Subtract : Sum  Inputs=+-
  Switch : Switch  Criteria=u2 > Threshold  ZeroCross=off  SaturateOnIntegerOverflow=off  InputSameDT=off
  increment : Constant  Value=0.2
  Joint 1 : Outport
  wires:
  Gain/1 -> Switch/3
  Subtract/1 -> Compare To Zero/1
  Compare To Zero/1 -> Switch/2
  Integrator/1 -> Joint 1/1, Subtract/1
  Switch/1 -> Integrator/1
  increment/1 -> Switch/1, Gain/1
  In1/1 -> Subtract/2

== system Hand/ApproachToAngle2/approacher1 ==
  In1 : Inport
  Compare To Zero : simulink/Logic and Bit Operations/Compare To Zero  relop=<=  OutDataTypeStr=boolean  ZeroCross=off
  Gain : Gain  Gain=-1
  Integrator : Integrator  ZeroCross=off
  Subtract : Sum  Inputs=+-
  Switch : Switch  Criteria=u2 > Threshold  ZeroCross=off  SaturateOnIntegerOverflow=off  InputSameDT=off
  increment : Constant  Value=0.2
  Joint 1 : Outport
  wires:
  Gain/1 -> Switch/3
  Subtract/1 -> Compare To Zero/1
  Compare To Zero/1 -> Switch/2
  Integrator/1 -> Joint 1/1, Subtract/1
  Switch/1 -> Integrator/1
  increment/1 -> Switch/1, Gain/1
  In1/1 -> Subtract/2

== system Hand/ApproachToAngle2/approacher2 ==
  In1 : Inport
  Compare To Zero : simulink/Logic and Bit Operations/Compare To Zero  relop=<=  OutDataTypeStr=boolean  ZeroCross=off
  Gain : Gain  Gain=-1
  Integrator : Integrator  ZeroCross=off
  Subtract : Sum  Inputs=+-
  Switch : Switch  Criteria=u2 > Threshold  ZeroCross=off  SaturateOnIntegerOverflow=off  InputSameDT=off
  increment : Constant  Value=0.2
  Joint 1 : Outport
  wires:
  Gain/1 -> Switch/3
  Subtract/1 -> Compare To Zero/1
  Compare To Zero/1 -> Switch/2
  Integrator/1 -> Joint 1/1, Subtract/1
  Switch/1 -> Integrator/1
  increment/1 -> Switch/1, Gain/1
  In1/1 -> Subtract/2

== system Hand/ApproachToAngle2/approacher3 ==
  In1 : Inport
  Compare To Zero : simulink/Logic and Bit Operations/Compare To Zero  relop=<=  OutDataTypeStr=boolean  ZeroCross=off
  Gain : Gain  Gain=-1
  Integrator : Integrator  ZeroCross=off
  Subtract : Sum  Inputs=+-
  Switch : Switch  Criteria=u2 > Threshold  ZeroCross=off  SaturateOnIntegerOverflow=off  InputSameDT=off
  increment : Constant  Value=0.2
  Joint 1 : Outport
  wires:
  Gain/1 -> Switch/3
  Subtract/1 -> Compare To Zero/1
  Compare To Zero/1 -> Switch/2
  Integrator/1 -> Joint 1/1, Subtract/1
  Switch/1 -> Integrator/1
  increment/1 -> Switch/1, Gain/1
  In1/1 -> Subtract/2

== system Hand/ApproachToAngle3/approacher1 ==
  In1 : Inport
  Compare To Zero : simulink/Logic and Bit Operations/Compare To Zero  relop=<=  OutDataTypeStr=boolean  ZeroCross=off
  Gain : Gain  Gain=-1
  Integrator : Integrator  ZeroCross=off
  Subtract : Sum  Inputs=+-
  Switch : Switch  Criteria=u2 > Threshold  ZeroCross=off  SaturateOnIntegerOverflow=off  InputSameDT=off
  increment : Constant  Value=0.2
  Joint 1 : Outport
  wires:
  Gain/1 -> Switch/3
  Subtract/1 -> Compare To Zero/1
  Compare To Zero/1 -> Switch/2
  Integrator/1 -> Joint 1/1, Subtract/1
  Switch/1 -> Integrator/1
  increment/1 -> Switch/1, Gain/1
  In1/1 -> Subtract/2

== system Hand/ApproachToAngle3/approacher2 ==
  In1 : Inport
  Compare To Zero : simulink/Logic and Bit Operations/Compare To Zero  relop=<=  OutDataTypeStr=boolean  ZeroCross=off
  Gain : Gain  Gain=-1
  Integrator : Integrator  ZeroCross=off
  Subtract : Sum  Inputs=+-
  Switch : Switch  Criteria=u2 > Threshold  ZeroCross=off  SaturateOnIntegerOverflow=off  InputSameDT=off
  increment : Constant  Value=0.2
  Joint 1 : Outport
  wires:
  Gain/1 -> Switch/3
  Subtract/1 -> Compare To Zero/1
  Compare To Zero/1 -> Switch/2
  Integrator/1 -> Joint 1/1, Subtract/1
  Switch/1 -> Integrator/1
  increment/1 -> Switch/1, Gain/1
  In1/1 -> Subtract/2

== system Hand/ApproachToAngle3/approacher3 ==
  In1 : Inport
  Compare To Zero : simulink/Logic and Bit Operations/Compare To Zero  relop=<=  OutDataTypeStr=boolean  ZeroCross=off
  Gain : Gain  Gain=-1
  Integrator : Integrator  ZeroCross=off
  Subtract : Sum  Inputs=+-
  Switch : Switch  Criteria=u2 > Threshold  ZeroCross=off  SaturateOnIntegerOverflow=off  InputSameDT=off
  increment : Constant  Value=0.2
  Joint 1 : Outport
  wires:
  Gain/1 -> Switch/3
  Subtract/1 -> Compare To Zero/1
  Compare To Zero/1 -> Switch/2
  Integrator/1 -> Joint 1/1, Subtract/1
  Switch/1 -> Integrator/1
  increment/1 -> Switch/1, Gain/1
  In1/1 -> Subtract/2

== system Hand/ApproachToAngle4/approacher1 ==
  In1 : Inport
  Compare To Zero : simulink/Logic and Bit Operations/Compare To Zero  relop=<=  OutDataTypeStr=boolean  ZeroCross=off
  Gain : Gain  Gain=-1
  Integrator : Integrator  ZeroCross=off
  Subtract : Sum  Inputs=+-
  Switch : Switch  Criteria=u2 > Threshold  ZeroCross=off  SaturateOnIntegerOverflow=off  InputSameDT=off
  increment : Constant  Value=0.2
  Joint 1 : Outport
  wires:
  Gain/1 -> Switch/3
  Subtract/1 -> Compare To Zero/1
  Compare To Zero/1 -> Switch/2
  Integrator/1 -> Joint 1/1, Subtract/1
  Switch/1 -> Integrator/1
  increment/1 -> Switch/1, Gain/1
  In1/1 -> Subtract/2

== system Hand/ApproachToAngle4/approacher2 ==
  In1 : Inport
  Compare To Zero : simulink/Logic and Bit Operations/Compare To Zero  relop=<=  OutDataTypeStr=boolean  ZeroCross=off
  Gain : Gain  Gain=-1
  Integrator : Integrator  ZeroCross=off
  Subtract : Sum  Inputs=+-
  Switch : Switch  Criteria=u2 > Threshold  ZeroCross=off  SaturateOnIntegerOverflow=off  InputSameDT=off
  increment : Constant  Value=0.2
  Joint 1 : Outport
  wires:
  Gain/1 -> Switch/3
  Subtract/1 -> Compare To Zero/1
  Compare To Zero/1 -> Switch/2
  Integrator/1 -> Joint 1/1, Subtract/1
  Switch/1 -> Integrator/1
  increment/1 -> Switch/1, Gain/1
  In1/1 -> Subtract/2

== system Hand/ApproachToAngle4/approacher3 ==
  In1 : Inport
  Compare To Zero : simulink/Logic and Bit Operations/Compare To Zero  relop=<=  OutDataTypeStr=boolean  ZeroCross=off
  Gain : Gain  Gain=-1
  Integrator : Integrator  ZeroCross=off
  Subtract : Sum  Inputs=+-
  Switch : Switch  Criteria=u2 > Threshold  ZeroCross=off  SaturateOnIntegerOverflow=off  InputSameDT=off
  increment : Constant  Value=0.2
  Joint 1 : Outport
  wires:
  Gain/1 -> Switch/3
  Subtract/1 -> Compare To Zero/1
  Compare To Zero/1 -> Switch/2
  Integrator/1 -> Joint 1/1, Subtract/1
  Switch/1 -> Integrator/1
  increment/1 -> Switch/1, Gain/1
  In1/1 -> Subtract/2

== system Hand/Subsystem1/Angle To Orientation ==
  Y : Inport
  X : Inport  Port=2
  Z : Inport  Port=3
  Multiplier3 : Constant  Value=-1
  Product : Product
  Rotation Angles : Concatenate  NumInputs=3  Mode=Multidimensional array
  Rotation Angles to Direction Cosine Matrix : sharedtransform/Rotation Angles to Direction Cosine Matrix  rotationOrder=XYZ  aMode=aMode
  Rotation Matrix to VR Rotation : vrlib/Utilities/Rotation Matrix to VR Rotation  maxzero=1e-12
  Out1 : Outport
  wires:
  Product/1 -> Rotation Angles to Direction Cosine Matrix/1
  Multiplier3/1 -> Product/1
  Y/1 -> Rotation Angles/2
  Rotation Angles to Direction Cosine Matrix/1 -> Rotation Matrix to VR Rotation/1
  Rotation Matrix to VR Rotation/1 -> Out1/1
  Rotation Angles/1 -> Product/2
  X/1 -> Rotation Angles/1
  Z/1 -> Rotation Angles/3

== system Hand/Subsystem1/Angle To Orientation1 ==
  Y : Inport
  X : Inport  Port=2
  Z : Inport  Port=3
  Multiplier3 : Constant  Value=-1
  Product : Product
  Rotation Angles : Concatenate  NumInputs=3  Mode=Multidimensional array
  Rotation Angles to Direction Cosine Matrix : sharedtransform/Rotation Angles to Direction Cosine Matrix  rotationOrder=XYZ  aMode=aMode
  Rotation Matrix to VR Rotation : vrlib/Utilities/Rotation Matrix to VR Rotation  maxzero=1e-12
  Out1 : Outport
  wires:
  Product/1 -> Rotation Angles to Direction Cosine Matrix/1
  Multiplier3/1 -> Product/1
  Y/1 -> Rotation Angles/2
  Rotation Angles to Direction Cosine Matrix/1 -> Rotation Matrix to VR Rotation/1
  Rotation Matrix to VR Rotation/1 -> Out1/1
  Rotation Angles/1 -> Product/2
  X/1 -> Rotation Angles/1
  Z/1 -> Rotation Angles/3

== system Hand/Subsystem1/Angle To Orientation2 ==
  Y : Inport
  X : Inport  Port=2
  Z : Inport  Port=3
  Multiplier3 : Constant  Value=-1
  Product : Product
  Rotation Angles : Concatenate  NumInputs=3  Mode=Multidimensional array
  Rotation Angles to Direction Cosine Matrix : sharedtransform/Rotation Angles to Direction Cosine Matrix  rotationOrder=XYZ  aMode=aMode
  Rotation Matrix to VR Rotation : vrlib/Utilities/Rotation Matrix to VR Rotation  maxzero=1e-12
  Out1 : Outport
  wires:
  Product/1 -> Rotation Angles to Direction Cosine Matrix/1
  Multiplier3/1 -> Product/1
  Y/1 -> Rotation Angles/2
  Rotation Angles to Direction Cosine Matrix/1 -> Rotation Matrix to VR Rotation/1
  Rotation Matrix to VR Rotation/1 -> Out1/1
  Rotation Angles/1 -> Product/2
  X/1 -> Rotation Angles/1
  Z/1 -> Rotation Angles/3

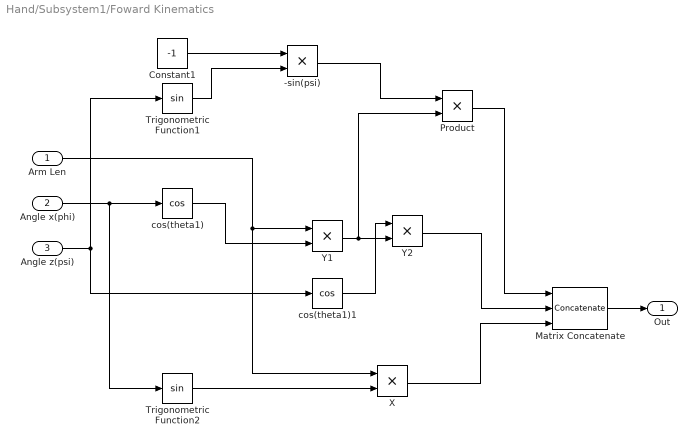
== system Hand/Subsystem1/Foward Kinematics ==
  Arm Len : Inport
  Angle x(phi) : Inport  Port=2
  Angle z(psi) : Inport  Port=3
  -sin(psi) : Product
  Constant1 : Constant  Value=-1
  Matrix Concatenate : Concatenate  NumInputs=3  ConcatenateDimension=2
  Product : Product
  Trigonometric Function1 : Trigonometry  OutputSignalType=real
  Trigonometric Function2 : Trigonometry  OutputSignalType=real
  X : Product
  Y1 : Product
  Y2 : Product
  cos(theta1) : Trigonometry  Operator=cos
  cos(theta1)1 : Trigonometry  Operator=cos
  Out : Outport
  wires:
  Matrix Concatenate/1 -> Out/1
  X/1 -> Matrix Concatenate/3
  Arm Len/1 -> X/1, Y1/1
  Trigonometric Function2/1 -> X/2
  Y1/1 -> Product/2, Y2/2
  cos(theta1)1/1 -> Y2/1
  Y2/1 -> Matrix Concatenate/2
  Product/1 -> Matrix Concatenate/1
  Constant1/1 -> -sin(psi)/1
  Trigonometric Function1/1 -> -sin(psi)/2
  Angle x(phi)/1 -> Trigonometric Function2/1, cos(theta1)/1
  cos(theta1)/1 -> Y1/2
  Angle z(psi)/1 -> Trigonometric Function1/1, cos(theta1)1/1
  -sin(psi)/1 -> Product/1

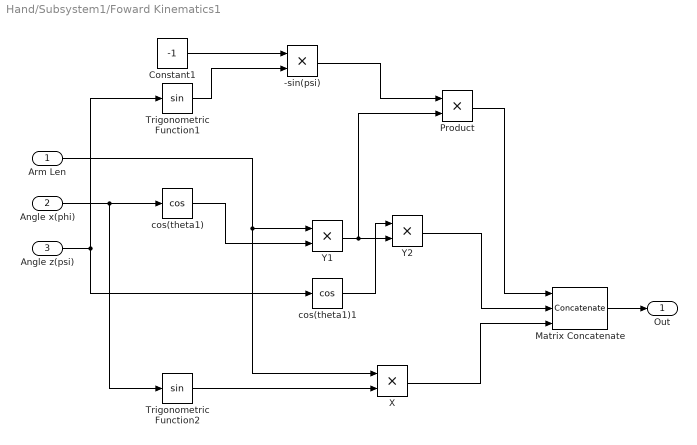
== system Hand/Subsystem1/Foward Kinematics1 ==
  Arm Len : Inport
  Angle x(phi) : Inport  Port=2
  Angle z(psi) : Inport  Port=3
  -sin(psi) : Product
  Constant1 : Constant  Value=-1
  Matrix Concatenate : Concatenate  NumInputs=3  ConcatenateDimension=2
  Product : Product
  Trigonometric Function1 : Trigonometry  OutputSignalType=real
  Trigonometric Function2 : Trigonometry  OutputSignalType=real
  X : Product
  Y1 : Product
  Y2 : Product
  cos(theta1) : Trigonometry  Operator=cos
  cos(theta1)1 : Trigonometry  Operator=cos
  Out : Outport
  wires:
  Matrix Concatenate/1 -> Out/1
  X/1 -> Matrix Concatenate/3
  Arm Len/1 -> X/1, Y1/1
  Trigonometric Function2/1 -> X/2
  Y1/1 -> Product/2, Y2/2
  cos(theta1)1/1 -> Y2/1
  Y2/1 -> Matrix Concatenate/2
  Product/1 -> Matrix Concatenate/1
  Constant1/1 -> -sin(psi)/1
  Trigonometric Function1/1 -> -sin(psi)/2
  Angle x(phi)/1 -> Trigonometric Function2/1, cos(theta1)/1
  cos(theta1)/1 -> Y1/2
  Angle z(psi)/1 -> Trigonometric Function1/1, cos(theta1)1/1
  -sin(psi)/1 -> Product/1

== system Hand/Subsystem2/Angle To Orientation ==
  Y : Inport
  X : Inport  Port=2
  Z : Inport  Port=3
  Multiplier3 : Constant  Value=-1
  Product : Product
  Rotation Angles : Concatenate  NumInputs=3  Mode=Multidimensional array
  Rotation Angles to Direction Cosine Matrix : sharedtransform/Rotation Angles to Direction Cosine Matrix  rotationOrder=XYZ  aMode=aMode
  Rotation Matrix to VR Rotation : vrlib/Utilities/Rotation Matrix to VR Rotation  maxzero=1e-12
  Out1 : Outport
  wires:
  Product/1 -> Rotation Angles to Direction Cosine Matrix/1
  Multiplier3/1 -> Product/1
  Y/1 -> Rotation Angles/2
  Rotation Angles to Direction Cosine Matrix/1 -> Rotation Matrix to VR Rotation/1
  Rotation Matrix to VR Rotation/1 -> Out1/1
  Rotation Angles/1 -> Product/2
  X/1 -> Rotation Angles/1
  Z/1 -> Rotation Angles/3

== system Hand/Subsystem2/Angle To Orientation1 ==
  Y : Inport
  X : Inport  Port=2
  Z : Inport  Port=3
  Multiplier3 : Constant  Value=-1
  Product : Product
  Rotation Angles : Concatenate  NumInputs=3  Mode=Multidimensional array
  Rotation Angles to Direction Cosine Matrix : sharedtransform/Rotation Angles to Direction Cosine Matrix  rotationOrder=XYZ  aMode=aMode
  Rotation Matrix to VR Rotation : vrlib/Utilities/Rotation Matrix to VR Rotation  maxzero=1e-12
  Out1 : Outport
  wires:
  Product/1 -> Rotation Angles to Direction Cosine Matrix/1
  Multiplier3/1 -> Product/1
  Y/1 -> Rotation Angles/2
  Rotation Angles to Direction Cosine Matrix/1 -> Rotation Matrix to VR Rotation/1
  Rotation Matrix to VR Rotation/1 -> Out1/1
  Rotation Angles/1 -> Product/2
  X/1 -> Rotation Angles/1
  Z/1 -> Rotation Angles/3

== system Hand/Subsystem2/Angle To Orientation2 ==
  Y : Inport
  X : Inport  Port=2
  Z : Inport  Port=3
  Multiplier3 : Constant  Value=-1
  Product : Product
  Rotation Angles : Concatenate  NumInputs=3  Mode=Multidimensional array
  Rotation Angles to Direction Cosine Matrix : sharedtransform/Rotation Angles to Direction Cosine Matrix  rotationOrder=XYZ  aMode=aMode
  Rotation Matrix to VR Rotation : vrlib/Utilities/Rotation Matrix to VR Rotation  maxzero=1e-12
  Out1 : Outport
  wires:
  Product/1 -> Rotation Angles to Direction Cosine Matrix/1
  Multiplier3/1 -> Product/1
  Y/1 -> Rotation Angles/2
  Rotation Angles to Direction Cosine Matrix/1 -> Rotation Matrix to VR Rotation/1
  Rotation Matrix to VR Rotation/1 -> Out1/1
  Rotation Angles/1 -> Product/2
  X/1 -> Rotation Angles/1
  Z/1 -> Rotation Angles/3

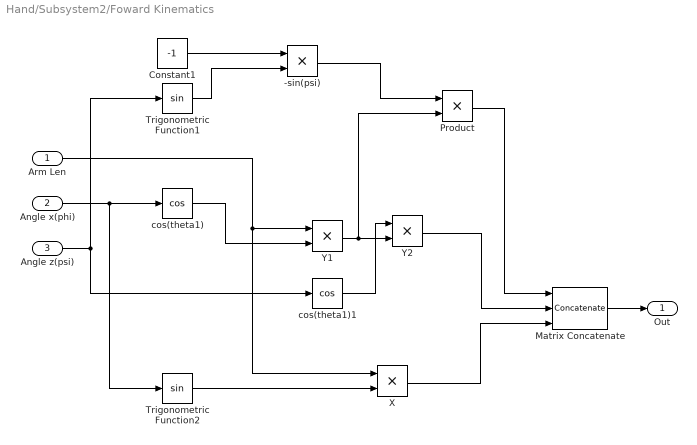
== system Hand/Subsystem2/Foward Kinematics ==
  Arm Len : Inport
  Angle x(phi) : Inport  Port=2
  Angle z(psi) : Inport  Port=3
  -sin(psi) : Product
  Constant1 : Constant  Value=-1
  Matrix Concatenate : Concatenate  NumInputs=3  ConcatenateDimension=2
  Product : Product
  Trigonometric Function1 : Trigonometry  OutputSignalType=real
  Trigonometric Function2 : Trigonometry  OutputSignalType=real
  X : Product
  Y1 : Product
  Y2 : Product
  cos(theta1) : Trigonometry  Operator=cos
  cos(theta1)1 : Trigonometry  Operator=cos
  Out : Outport
  wires:
  Matrix Concatenate/1 -> Out/1
  X/1 -> Matrix Concatenate/3
  Arm Len/1 -> X/1, Y1/1
  Trigonometric Function2/1 -> X/2
  Y1/1 -> Product/2, Y2/2
  cos(theta1)1/1 -> Y2/1
  Y2/1 -> Matrix Concatenate/2
  Product/1 -> Matrix Concatenate/1
  Constant1/1 -> -sin(psi)/1
  Trigonometric Function1/1 -> -sin(psi)/2
  Angle x(phi)/1 -> Trigonometric Function2/1, cos(theta1)/1
  cos(theta1)/1 -> Y1/2
  Angle z(psi)/1 -> Trigonometric Function1/1, cos(theta1)1/1
  -sin(psi)/1 -> Product/1

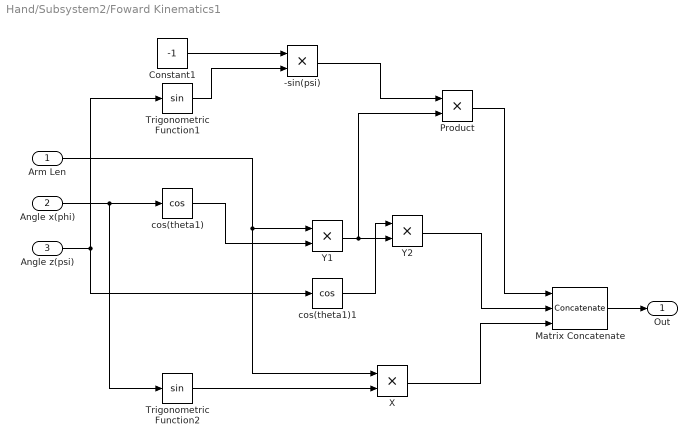
== system Hand/Subsystem2/Foward Kinematics1 ==
  Arm Len : Inport
  Angle x(phi) : Inport  Port=2
  Angle z(psi) : Inport  Port=3
  -sin(psi) : Product
  Constant1 : Constant  Value=-1
  Matrix Concatenate : Concatenate  NumInputs=3  ConcatenateDimension=2
  Product : Product
  Trigonometric Function1 : Trigonometry  OutputSignalType=real
  Trigonometric Function2 : Trigonometry  OutputSignalType=real
  X : Product
  Y1 : Product
  Y2 : Product
  cos(theta1) : Trigonometry  Operator=cos
  cos(theta1)1 : Trigonometry  Operator=cos
  Out : Outport
  wires:
  Matrix Concatenate/1 -> Out/1
  X/1 -> Matrix Concatenate/3
  Arm Len/1 -> X/1, Y1/1
  Trigonometric Function2/1 -> X/2
  Y1/1 -> Product/2, Y2/2
  cos(theta1)1/1 -> Y2/1
  Y2/1 -> Matrix Concatenate/2
  Product/1 -> Matrix Concatenate/1
  Constant1/1 -> -sin(psi)/1
  Trigonometric Function1/1 -> -sin(psi)/2
  Angle x(phi)/1 -> Trigonometric Function2/1, cos(theta1)/1
  cos(theta1)/1 -> Y1/2
  Angle z(psi)/1 -> Trigonometric Function1/1, cos(theta1)1/1
  -sin(psi)/1 -> Product/1

== system Hand/Subsystem3/Angle To Orientation ==
  Y : Inport
  X : Inport  Port=2
  Z : Inport  Port=3
  Multiplier3 : Constant  Value=-1
  Product : Product
  Rotation Angles : Concatenate  NumInputs=3  Mode=Multidimensional array
  Rotation Angles to Direction Cosine Matrix : sharedtransform/Rotation Angles to Direction Cosine Matrix  rotationOrder=XYZ  aMode=aMode
  Rotation Matrix to VR Rotation : vrlib/Utilities/Rotation Matrix to VR Rotation  maxzero=1e-12
  Out1 : Outport
  wires:
  Product/1 -> Rotation Angles to Direction Cosine Matrix/1
  Multiplier3/1 -> Product/1
  Y/1 -> Rotation Angles/2
  Rotation Angles to Direction Cosine Matrix/1 -> Rotation Matrix to VR Rotation/1
  Rotation Matrix to VR Rotation/1 -> Out1/1
  Rotation Angles/1 -> Product/2
  X/1 -> Rotation Angles/1
  Z/1 -> Rotation Angles/3
